simulink model "Problem2"  (R2020a)
settings: Solver=VariableStepAuto  StartTime=0.0  StopTime=10.0  RelTol=1e-3
model workspace (MAT data in the model file):
  B = 1
  Ks = 1
  Kw = 1
  M1 = 1
  M2 = 1
settings Model: OrderedModelArguments=off  Creator=tnradm  LastModifiedBy=tnradm

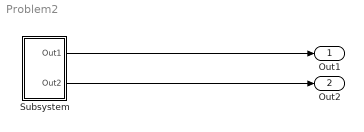
== system Problem2 ==
  Subsystem : Subsystem  mask{M1=1, M2=1, Ks=1, Kw=1, B=1}
  Out1 : Outport
  Out2 : Outport  Port=2
  wires:
  Subsystem/1(Out1) -> Out1/1
  Subsystem/2(Out2) -> Out2/1

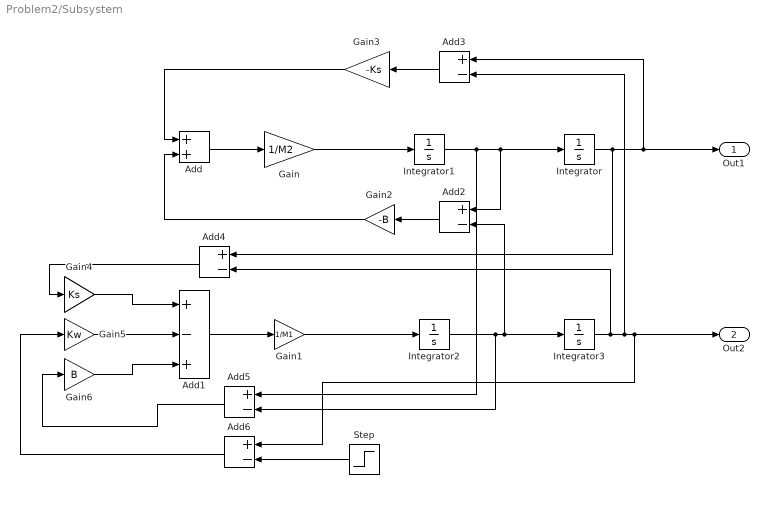
== system Problem2/Subsystem ==
  Add : Sum
  Add1 : Sum  Inputs=+-+
  Add{2..6} (5 alike) : Sum  Inputs=+-
  Gain : Gain  Gain=1/M2
  Gain1 : Gain  Gain=1/M1
  Gain2 : Gain  Gain=-B
  Gain3 : Gain  Gain=-Ks
  Gain4 : Gain  Gain=Ks
  Gain5 : Gain  Gain=Kw
  Gain6 : Gain  Gain=B
  Integrator{,1..3} (4 alike) : Integrator
  Step : Step  SampleTime=0
  Out1 : Outport
  Out2 : Outport  Port=2
  wires:
  Gain1/1 -> Integrator2/1
  Integrator1/1 -> Add5/1, Add2/1, Integrator/1
  Gain4/1 -> Add1/1
  Integrator/1 -> Add4/1, Out1/1, Add3/1
  Integrator2/1 -> Add2/2, Integrator3/1, Add5/2
  Add/1 -> Gain/1
  Integrator3/1 -> Add4/2, Add3/2, Out2/1, Add6/1
  Step/1 -> Add6/2
  Gain6/1 -> Add1/3
  Gain3/1 -> Add/1
  Add5/1 -> Gain6/1
  Add6/1 -> Gain5/1
  Gain5/1 -> Add1/2
  Add3/1 -> Gain3/1
  Gain/1 -> Integrator1/1
  Add1/1 -> Gain1/1
  Add4/1 -> Gain4/1
  Add2/1 -> Gain2/1
  Gain2/1 -> Add/2
